simulink model "return_journey"  (R2016a)
settings: Solver=FixedStepAuto  StartTime=Param.T  StopTime=Param.TStop  FixedStep=Param.deltaT  RelTol=1e-3
undefined symbols (not defined in the file or in its folder): controlVec, drawRetPath, neuralNetwork, Param, stopSim, updateRetPosn, X, Y, Z
libraries: robotlib x6
settings Model: Creator=Emily  LastModifiedBy=Emily

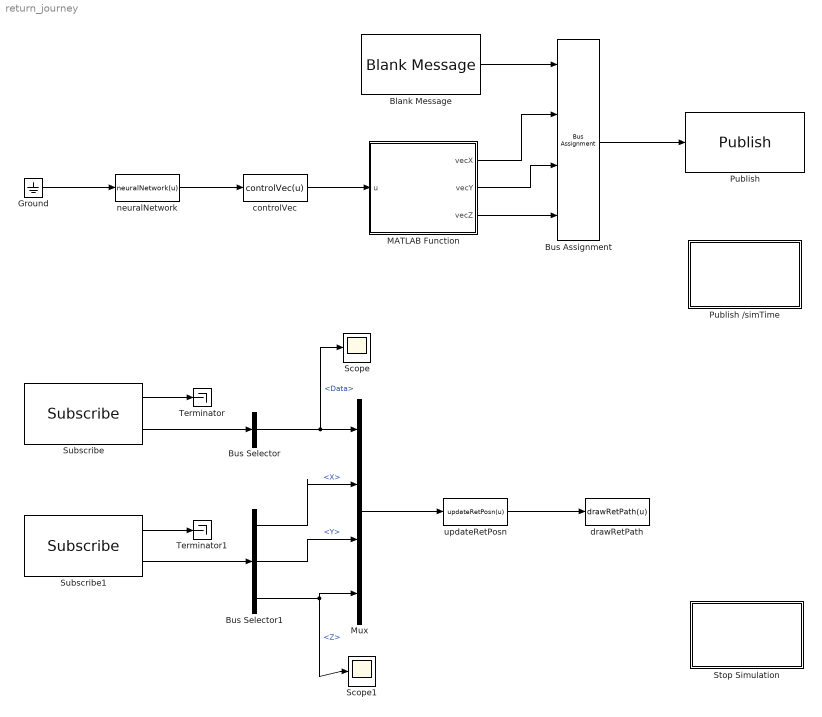
== system return_journey ==
  Blank Message : robotlib/Blank Message  SourceLibraryInfo=This block requires Robotics System Toolbox  messageType=geometry_msgs/Vector3  SampleTime=inf
  Bus Assignment : BusAssignment  AssignedSignals=X,Y,Z
  Bus Selector : BusSelector  OutputSignals=Data
  Bus Selector1 : BusSelector  OutputSignals=X,Y,Z
  Ground : Ground
  MATLAB Function : MATLAB Function  TreatAsAtomicUnit=on
  Mux : Mux  Inputs=[1 1 1 1]
  Publish : robotlib/Publish  SourceLibraryInfo=This block requires Robotics System Toolbox  topicSource=Specify your own  topic=/simDir  messageType=geometry_msgs/Vector3  messageQueueLength=1
  Publish /simTime : Subsystem
  Scope : Scope
  Scope1 : Scope
  Stop Simulation : Subsystem
  Subscribe : robotlib/Subscribe  SourceLibraryInfo=This block requires Robotics System Toolbox  topicSource=Specify your own  topic=/simTime  messageType=std_msgs/Float64  sampleTime=-1  messageQueueLength=1
  Subscribe1 : robotlib/Subscribe  SourceLibraryInfo=This block requires Robotics System Toolbox  topicSource=Specify your own  topic=/simDir  messageType=geometry_msgs/Vector3  sampleTime=-1  messageQueueLength=1
  Terminator : Terminator
  Terminator1 : Terminator
  controlVec : MATLABFcn  MATLABFcn=controlVec(u)  OutputDimensions=3
  drawRetPath : MATLABFcn  MATLABFcn=drawRetPath(u)  OutputDimensions=0
  neuralNetwork : MATLABFcn  MATLABFcn=neuralNetwork(u)  OutputDimensions=8
  updateRetPosn : MATLABFcn  MATLABFcn=updateRetPosn(u)  OutputDimensions=4
  wires:
  neuralNetwork/1 -> controlVec/1
  Ground/1 -> neuralNetwork/1
  controlVec/1 -> MATLAB Function/1(u)
  Blank Message/1 -> Bus Assignment/1
  MATLAB Function/1(vecX) -> Bus Assignment/2
  MATLAB Function/2(vecY) -> Bus Assignment/3
  MATLAB Function/3(vecZ) -> Bus Assignment/4
  Bus Assignment/1 -> Publish/1
  Subscribe1/1 -> Terminator1/1
  Subscribe/1 -> Terminator/1
  Subscribe1/2 -> Bus Selector1/1
  Subscribe/2 -> Bus Selector/1
  Bus Selector/1 -> Scope/1, Mux/1  "<Data>"
  Bus Selector1/1 -> Mux/2  "<X>"
  Bus Selector1/2 -> Mux/3  "<Y>"
  Bus Selector1/3 -> Scope1/1, Mux/4  "<Z>"
  Mux/1 -> updateRetPosn/1
  updateRetPosn/1 -> drawRetPath/1

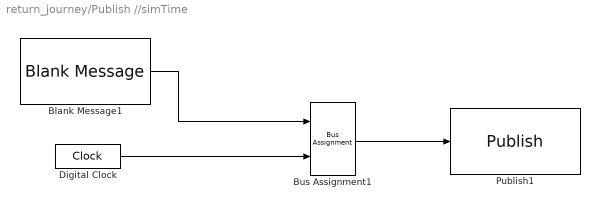
== system return_journey/Publish //simTime ==
  Blank Message1 : robotlib/Blank Message  SourceLibraryInfo=This block requires Robotics System Toolbox  messageType=std_msgs/Float64  SampleTime=inf
  Bus Assignment1 : BusAssignment  AssignedSignals=Data
  Digital Clock : DigitalClock  SampleTime=Param.deltaT
  Publish1 : robotlib/Publish  SourceLibraryInfo=This block requires Robotics System Toolbox  topicSource=Specify your own  topic=/simTime  messageType=std_msgs/Float64  messageQueueLength=1
  wires:
  Digital Clock/1 -> Bus Assignment1/2
  Bus Assignment1/1 -> Publish1/1
  Blank Message1/1 -> Bus Assignment1/1

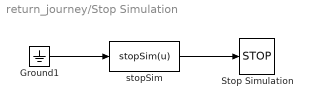
== system return_journey/Stop Simulation ==
  Ground1 : Ground
  Stop Simulation : Stop
  stopSim : MATLABFcn  MATLABFcn=stopSim(u)
  wires:
  stopSim/1 -> Stop Simulation/1
  Ground1/1 -> stopSim/1

== matlab function return_journey/MATLAB Function ==
  data: u input; vecX output; vecY output; vecZ output
% returns the individual elements of the dirV vector
% inputs:
%   u, a 3x1 vector (dirV)
% outputs:
%   vecX, the x element of dirV
%   vecY, the y element of dirV
%   vecZ, the z element of dirV

function [vecX,vecY,vecZ] = dirVels(u)

    vecX = u(1);
    vecY = u(2);
    vecZ = u(3);
    
end
